simulink model "Mod5_Counter"  (R2020a)
settings: Solver=VariableStepAuto  StartTime=0.0  StopTime=inf  RelTol=1e-3
settings Model: Creator=Hp  LastModifiedBy=Hp

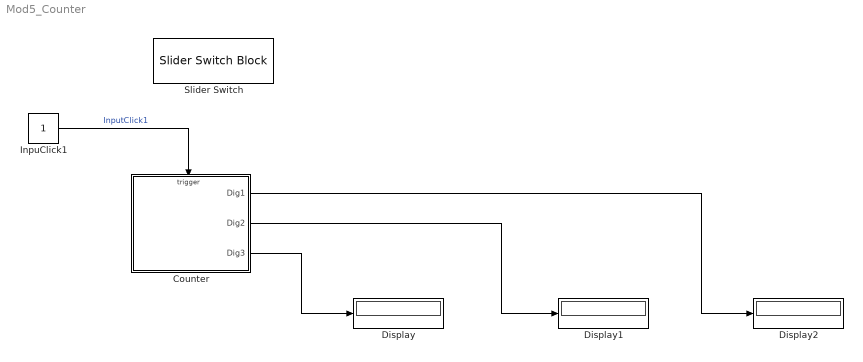
== system Mod5_Counter ==
  Counter : Stateflow chart  TreatAsAtomicUnit=on
  Display : Display
  Display1 : Display
  Display2 : Display
  InpuClick1 : Constant
  Slider Switch : SliderSwitchBlock
      settings: Values={{'Off', 'On'}, [0 1]}
  wires:
  InpuClick1/1 -> Counter/Trigger  "InputClick1"
  Counter/3(Dig3) -> Display/1
  Counter/2(Dig2) -> Display1/1
  Counter/1(Dig1) -> Display2/1

== stateflow chart Mod5_Counter/Counter ==
  state Digit1 [parallel]
    settings: executionOrder=1
    state Zero
      en:
      Dig1=0;
    state One
      en:
      Dig1=1;
    state Two
      en:
      Dig1=2;
    state Three
      en:
      Dig1=3;
    state Four
      en:
      Dig1=4;
    (default) -> Digit1.Zero
    Digit1.Zero -> Digit1.One : InputClick1
    Digit1.One -> Digit1.Two : InputClick1
    Digit1.Two -> Digit1.Three : InputClick1
    Digit1.Three -> Digit1.Four : InputClick1
    Digit1.Four -> Digit1.Zero : InputClick1/{InputClick2}
  state Digit2 [parallel]
    settings: executionOrder=2
    state Zero
      en:
      Dig2=0;
    state One
      en:
      Dig2=1;
    state Two
      en:
      Dig2=2;
    state Three
      en:
      Dig2=3;
    state Four
      en:
      Dig2=4;
    (default) -> Digit2.Zero
    Digit2.Zero -> Digit2.One : InputClick2
    Digit2.One -> Digit2.Two : InputClick2
    Digit2.Two -> Digit2.Three : InputClick2
    Digit2.Three -> Digit2.Four : InputClick2
    Digit2.Four -> Digit2.Zero : InputClick2/{InputClick3}
  state Digit3 [parallel]
    settings: executionOrder=3
    state Zero
      en:
      Dig3=0;
    state One
      en:
      Dig3=1;
    state Two
      en:
      Dig3=2;
    state Three
      en:
      Dig3=3;
    state Four
      en:
      Dig3=4;
    (default) -> Digit3.Zero
    Digit3.Zero -> Digit3.One : InputClick3
    Digit3.One -> Digit3.Two : InputClick3
    Digit3.Two -> Digit3.Three : InputClick3
    Digit3.Three -> Digit3.Four : InputClick3
    Digit3.Four -> Digit3.Zero : InputClick3
  data: Dig1 output; Dig2 output; Dig3 output
  events: InputClick2 local FUNCTION_CALL_EVENT; InputClick3 local RISING_EDGE_EVENT; InputClick1 input RISING_EDGE_EVENT
